simulink model "Bahn_uebergang"  (R2024b)
settings: Solver=VariableStepAuto  StartTime=0.0  StopTime=inf  RelTol=1e-3
settings Model: Creator=Steve Kinfack  LastModifiedBy=Steve Kinfack

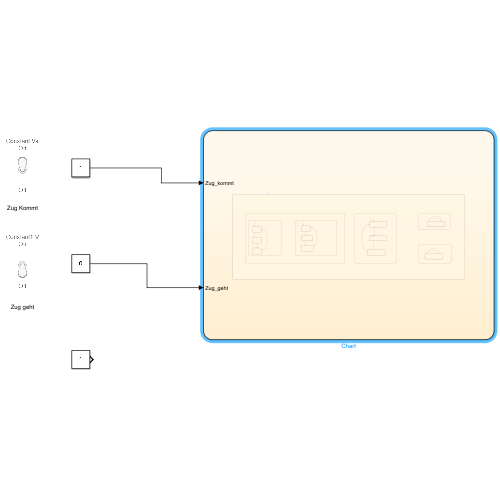
[thumbnail: Simulink's stored preview of the top-level diagram]
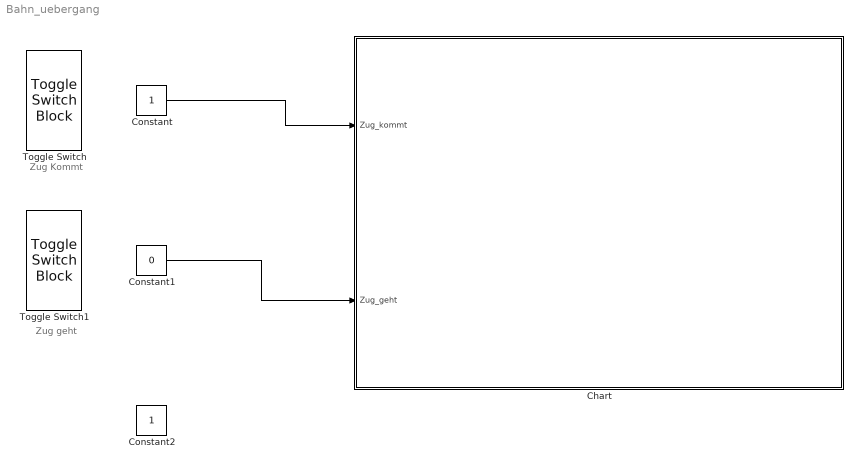
== system Bahn_uebergang ==
  note: Zug geht
  note: Zug Kommt
  Chart : Stateflow chart  TreatAsAtomicUnit=on
  Constant : Constant
  Constant1 : Constant  Value=0
  Constant2 : Constant
  Toggle Switch : ToggleSwitchBlock
      settings: Values={{'Off', 'On'}, [0 1]}
  Toggle Switch1 : ToggleSwitchBlock
      settings: Values={{'Off', 'On'}, [0 1]}
  wires:
  Constant/1 -> Chart/1(Zug_kommt)
  Constant1/1 -> Chart/2(Zug_geht)

== stateflow chart Bahn_uebergang/Chart ==
  settings: executeAtInitialization=1
  state Bahn_uebergang
    state Schranke [parallel]
      settings: executionOrder=2
      state S2 [parallel]
        settings: executionOrder=1
        state S2_Offen
        state delayS1_und_blink
        state S2_Zu
        (default) -> S2_Offen
        S2_Zu -> S2_Offen : [counter < 0 || counter == 0]
        S2_Offen -> delayS1_und_blink : [counter > 0]
        delayS1_und_blink -> S2_Zu : after(20, sec)
      state S1 [parallel]
        settings: executionOrder=2
        state S1_Offen
        state delay_blink
        state S1_Zu
        (default) -> S1_Offen
        S1_Zu -> S1_Offen : [counter < 0 || counter == 0]
        S1_Offen -> delay_blink : [counter > 0]
        delay_blink -> S1_Zu : after(10, sec)
    state Warnlich [parallel]
      settings: executionOrder=1
      state Warnlich_Aus
      state Warnlich_Blink
        Warnlich_Blink -> Warnlich_Blink [order 1]
      state Warnlich_rot
      (default) -> Warnlich_Aus
      Warnlich_rot -> Warnlich_Aus : [counter < 0 || counter == 0]
      Warnlich_Aus -> Warnlich_Blink : [counter > 0]
      Warnlich_Blink -> Warnlich_rot [order 1] : after(20, sec)
    state a [parallel]
      settings: executionOrder=3
      state zug_kommt
        entry: counter = counter + 1;
      zug_kommt -> zug_kommt : [Zug_kommt]
    state a1 [parallel]
      settings: executionOrder=4
      state zug_geht
        entry: counter = counter - 1;
      zug_geht -> zug_geht : [counter > 0 && Zug_geht ]
  (default) -> Bahn_uebergang
  data: counter local =0; Zug_kommt input; Zug_geht input
